simulink model "Test_ALU"  (Simulink 8.1)
settings: Solver=ode45  StartTime=0.0  StopTime=20.0  RelTol=1e-3
libraries: Computer_Library x1, simulink_extras x1
settings Model: Creator=uzivatel  LastModifiedBy=uzivatel
settings DataIOCC: SignalLoggingSaveFormat=Dataset
settings OptimizationCC: ExpressionDepthLimit=128
settings DebuggingCC: FcnCallInpInsideContextMsg=EnableAllAsError
settings GRTTargetCC: CombineOutputUpdateFcns=on  GRTInterface=off

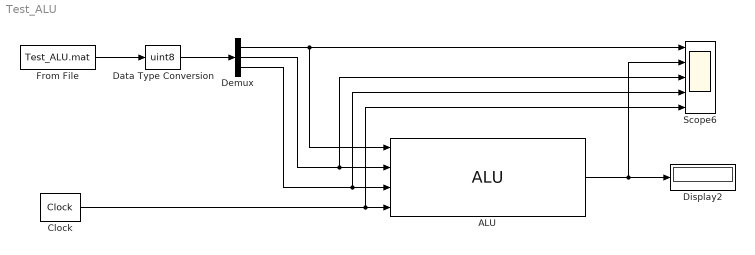
== system Test_ALU ==
  ALU : Computer_Library/ALU
  Clock : simulink_extras/Flip Flops/Clock  period=1
  Data Type Conversion : DataTypeConversion  OutDataTypeStr=uint8
  Demux : Demux  Outputs=3
  Display2 : Display
  From File : FromFile  FileName=Test_ALU.mat  OutDataTypeStr=double  SampleTime=1  ExtrapolationBeforeFirstDataPoint=Hold first value  ExtrapolationAfterLastDataPoint=Ground value
  Scope6 : Scope  NumInputPorts=5
      settings: YMin=0~0~0~0~0  YMax=255~255~1.5~3~1.5
  wires:
  Demux/2 -> ALU/2, Scope6/3
  Demux/1 -> ALU/1, Scope6/1
  Clock/1 -> ALU/4, Scope6/5
  ALU/1 -> Scope6/2, Display2/1
  Demux/3 -> Scope6/4, ALU/3
  From File/1 -> Data Type Conversion/1
  Data Type Conversion/1 -> Demux/1
